simulink model "VFsimplifiee_fonctionneMal"  (R2021b)
settings: Solver=ode15s  StartTime=0.0  StopTime=1500  RelTol=1e-3
settings Model: Creator=elina  LastModifiedBy=elina

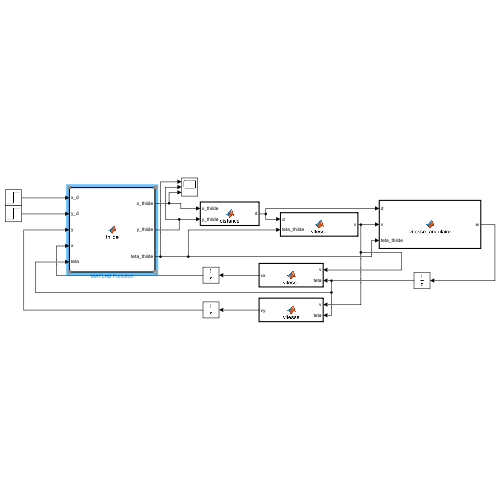
[thumbnail: Simulink's stored preview of the top-level diagram]
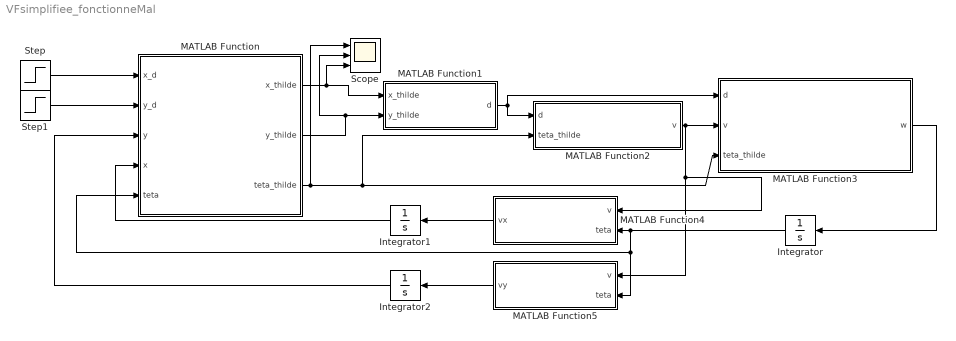
== system VFsimplifiee_fonctionneMal ==
  Integrator : Integrator
  Integrator1 : Integrator
  Integrator2 : Integrator
  MATLAB Function : MATLAB Function  TreatAsAtomicUnit=on
  MATLAB Function1 : MATLAB Function  TreatAsAtomicUnit=on
  MATLAB Function2 : MATLAB Function  TreatAsAtomicUnit=on
  MATLAB Function3 : MATLAB Function  TreatAsAtomicUnit=on
  MATLAB Function4 : MATLAB Function  TreatAsAtomicUnit=on
  MATLAB Function5 : MATLAB Function  TreatAsAtomicUnit=on
  Scope : Scope  NumInputPorts=3
  Step : Step  Time=0  After=10  SampleTime=0
  Step1 : Step  Time=0  After=10  SampleTime=0
  wires:
  MATLAB Function3/1(w) -> Integrator/1
  MATLAB Function/3(teta_thilde) -> MATLAB Function2/2(teta_thilde), MATLAB Function3/3(teta_thilde), Scope/1
  MATLAB Function/2(y_thilde) -> MATLAB Function1/2(y_thilde), Scope/2
  MATLAB Function/1(x_thilde) -> MATLAB Function1/1(x_thilde), Scope/3
  Step/1 -> MATLAB Function/1(x_d)
  Step1/1 -> MATLAB Function/2(y_d)
  Integrator/1 -> MATLAB Function5/2(teta), MATLAB Function/5(teta), MATLAB Function4/2(teta)
  MATLAB Function4/1(vx) -> Integrator1/1
  Integrator2/1 -> MATLAB Function/3(y)
  MATLAB Function5/1(vy) -> Integrator2/1
  Integrator1/1 -> MATLAB Function/4(x)
  MATLAB Function1/1(d) -> MATLAB Function3/1(d), MATLAB Function2/1(d)
  MATLAB Function2/1(v) -> MATLAB Function5/1(v), MATLAB Function4/1(v), MATLAB Function3/2(v)

== matlab function VFsimplifiee_fonctionneMal/MATLAB Function4 ==
  data: v input; vx output; teta input
function vx  =vitesse(v,teta)
vx=v*cos(teta);
end

== matlab function VFsimplifiee_fonctionneMal/MATLAB Function5 ==
  data: v input; vy output; teta input
function vy  =vitesse(v,teta)
vy=v*sin(teta);
end

== matlab function VFsimplifiee_fonctionneMal/MATLAB Function ==
  data: x_d input; x_thilde output; y_d input; y input; x input; teta input; y_thilde output; teta_thilde output
function [x_thilde,y_thilde,teta_thilde]=thilde(x_d,y_d,y,x,teta)
x_thilde=x_d-x;
y_thilde=y_d-y;
%teta=atan2(sin(teta),cos(teta));
teta_thilde=atan2(y_thilde,x_thilde)-teta;
%teta_thilde=atan2(y_thilde,x_thilde);
end

== matlab function VFsimplifiee_fonctionneMal/MATLAB Function1 ==
  data: x_thilde input; d output; y_thilde input
function d  =distance(x_thilde,y_thilde)
d=(x_thilde*x_thilde+y_thilde*y_thilde)^(1/2);
end

== matlab function VFsimplifiee_fonctionneMal/MATLAB Function2 ==
  data: d input; v output; teta_thilde input
function v  =vitesse(d,teta_thilde)
k1=0.5;
k3=2;
v_max=0.32;
v=abs((d/(k1+d))*v_max*cos(k3*teta_thilde));
end

== matlab function VFsimplifiee_fonctionneMal/MATLAB Function3 ==
  data: d input; v input; w output; teta_thilde input
function w  =vitesse_angulaire(d,v,teta_thilde)
k2=1;
k3=1;
if d<0.01
    w=(v/0.01)*sin(teta_thilde)+k2*tanh(k3*teta_thilde);

else
    w=(v/d)*sin(teta_thilde)+k2*tanh(k3*teta_thilde);
end
end
